simulink model "ACC_CarSim"  (Simulink 8.1)
settings: Solver=FixedStepDiscrete  StartTime=0.0  StopTime=100  FixedStep=0.001  MaxStep=0.001  RelTol=1e-3
PreLoadFcn:
  | Ts = 0.01;
undefined symbols (not defined in the file): DiscIntNeverNeededParam, sigbuilder_block
libraries: simulink x4, Solver_SF x1
settings Model: Creator=IVDL_Mola  LastModifiedBy=IVDL
settings DataIOCC: SignalLoggingSaveFormat=Dataset
settings OptimizationCC: ExpressionDepthLimit=128
settings DebuggingCC: FcnCallInpInsideContextMsg=EnableAllAsError  StateNameClashWarn=none
settings GRTTargetCC: CodeReplacementLibrary=None  CombineOutputUpdateFcns=on  CPPClassGenCompliant=on  GRTInterface=off

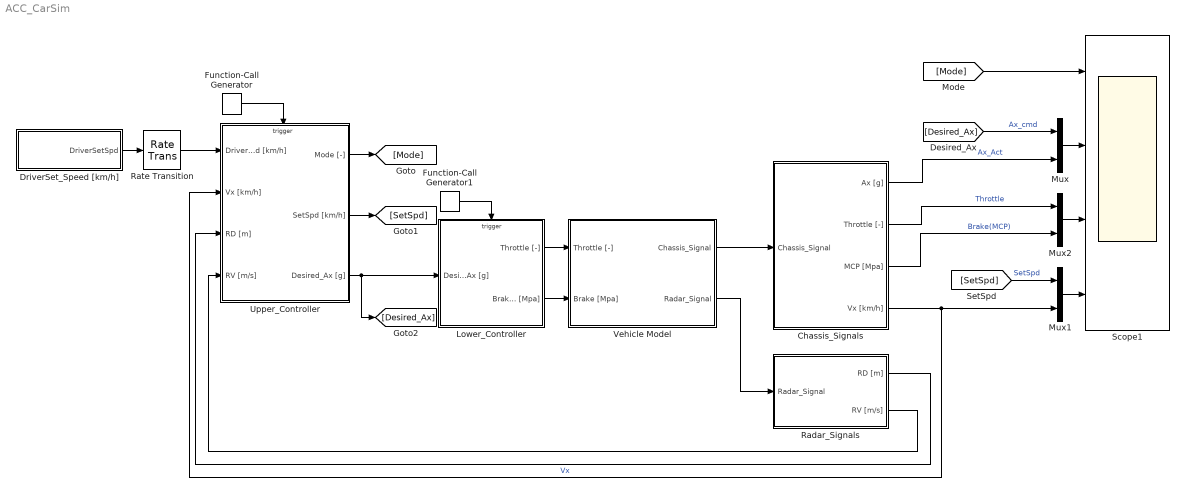
== system ACC_CarSim ==
  Chassis_Signals : Subsystem  SystemSampleTime=Ts
      settings: MinAlgLoopOccurrences=on
  DriverSet_Speed [km/h] : Subsystem  Tag=STV Subsys  LoadFcn=sigbuilder_block('load');  StartFcn=sigbuilder_block('start');  StopFcn=sigbuilder_block('stop');  ClipboardFcn=sigbuilder_block('clipboard');  mask(Sigbuilder block){}
      mask help: Simulink:masks:SigbuilderBlock_MD
      mask init:
      | if ~strcmp(get_param(bdroot(gcbh),'SimulationStatus'),'stopped') tuvar = sigbuilder_block('maskInit'); end
      settings: CopyFcn=sigbuilder_block('copy');  DeleteFcn=sigbuilder_block('delete');  ModelCloseFcn=sigbuilder_block('modelClose');  PreSaveFcn=sigbuilder_block('preSave');  PauseFcn=sigbuilder_block('pause');  ContinueFcn=sigbuilder_block('continue');  NameChangeFcn=sigbuilder_block('namechange');  OpenFcn=sigbuilder_block('open',[361.5 171.75 518.25 401.25 ]);  CloseFcn=sigbuilder_block('close');
      mask Display: plot(0, 0, 100, 100,[2, 2, 32, 32, 2], [68, 8, 8, 68, 68],[32, 2], [38, 38], [32, 19, 2],[53, 60, 44], [32, 17, 17, 2],[16, 16, 31, 31]);txt = getActiveGroup(gcbh);text(2, 100, txt,'verticalAlignment', 'top');
  Function-Call Generator : simulink/Ports & Subsystems/Function-Call Generator  sample_time=Ts  numberOfIterations=1
  Function-Call Generator1 : simulink/Ports & Subsystems/Function-Call Generator  sample_time=Ts  numberOfIterations=1
  Lower_Controller : Subsystem
  Mux : Mux  Inputs=2
  Mux1 : Mux  Inputs=2
  Mux2 : Mux  Inputs=2
  Radar_Signals : Subsystem  SystemSampleTime=Ts
  Rate Transition : RateTransition
  Scope1 : Scope  NumInputPorts=4
      settings: ShowLegends=on  TimeRange=100  YMin=0~-0.4~0~55  YMax=1~0.3~1.3~115
  Upper_Controller : Subsystem
  Vehicle Model : Subsystem
  wires:
  Upper_Controller/3(Desired_Ax [g]) -> [Desired_Ax], Lower_Controller/1(Desired_Ax [g])
  Lower_Controller/2(Brake [Mpa]) -> Vehicle Model/2(Brake [Mpa])
  Function-Call Generator/1 -> Upper_Controller/Trigger
  Function-Call Generator1/1 -> Lower_Controller/Trigger
  Vehicle Model/1(Chassis_Signal) -> Chassis_Signals/1(Chassis_Signal)
  Vehicle Model/2(Radar_Signal) -> Radar_Signals/1(Radar_Signal)
  Radar_Signals/2(RV [m/s]) -> Upper_Controller/4(RV [m/s])
  Radar_Signals/1(RD [m]) -> Upper_Controller/3(RD [m])
  DriverSet_Speed [km/h]/1(DriverSetSpd) -> Rate Transition/1
  Upper_Controller/1(Mode [-]) -> [Mode]
  Upper_Controller/2(SetSpd [km/h]) -> [SetSpd]
  Mux/1 -> Scope1/2
  Chassis_Signals/4(Vx [km/h]) -> Mux1/2, Upper_Controller/2(Vx [km/h])  "Vx"
  [Mode] -> Scope1/1
  [SetSpd] -> Mux1/1  "SetSpd"
  [Desired_Ax] -> Mux/1  "Ax_cmd"
  Mux2/1 -> Scope1/3
  Mux1/1 -> Scope1/4
  Chassis_Signals/1(Ax [g]) -> Mux/2  "Ax_Act"
  Chassis_Signals/2(Throttle [-]) -> Mux2/1  "Throttle"
  Chassis_Signals/3(MCP [Mpa]) -> Mux2/2  "Brake(MCP)"
  Rate Transition/1 -> Upper_Controller/1(Driver_SetSpd [km/h])
  Lower_Controller/1(Throttle [-]) -> Vehicle Model/1(Throttle [-])

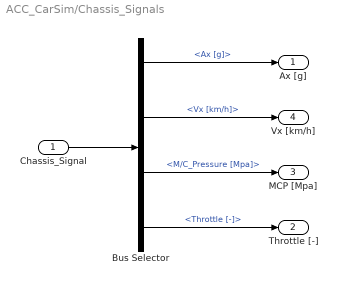
== system ACC_CarSim/Chassis_Signals ==
  Chassis_Signal : Inport
  Bus Selector : BusSelector  OutputSignals=Ax [g],Vx [km/h],M/C_Pressure [Mpa],Throttle [-]
  Ax [g] : Outport
  Throttle [-] : Outport  Port=2
  MCP [Mpa] : Outport  Port=3
  Vx [km/h] : Outport  Port=4
  wires:
  Bus Selector/2 -> Vx [km/h]/1  "<Vx [km/h]>"
  Bus Selector/1 -> Ax [g]/1  "<Ax [g]>"
  Chassis_Signal/1 -> Bus Selector/1
  Bus Selector/3 -> MCP [Mpa]/1  "<M/C_Pressure [Mpa]>"
  Bus Selector/4 -> Throttle [-]/1  "<Throttle [-]>"

== system ACC_CarSim/DriverSet_Speed [km/h] ==
  Demux : Demux  Tag=STV Demux  Outputs=1
  FromWs : FromWorkspace  Tag=STV FromWs  VariableName=tuvar  SampleTime=0  SigBuilderData=DataTag0  VnvData=DataTag1
      SigBuilderData=|
      | common.afterFinalStr = 'Extrapolate'
      | common.sampleTime = 0
      | dataSet.timeRange = [0 100]
      | dataSet.name = 'Group 1'
      | sbobj.Groups.Name = 'Group 1'
      | sbobj.Groups.Signals.Name = 'DriverSetSpd'
      | sbobj.Groups.Signals.XData = [0 25 25 80 80 100]
      | sbobj.Groups.Signals.YData = [70 70 110 110 60 60]
      | sbobj.Groups.TimeRange = [0 100]
  DriverSetSpd : Outport  Tag=STV Outport
  wires:
  Demux/1 -> DriverSetSpd/1
  FromWs/1 -> Demux/1

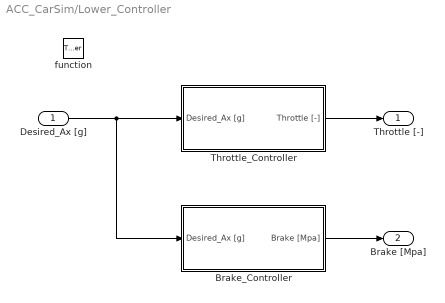
== system ACC_CarSim/Lower_Controller ==
  Desired_Ax [g] : Inport
  function : TriggerPort  TriggerType=function-call
  Brake_Controller : Subsystem
  Throttle_Controller : Subsystem
  Throttle [-] : Outport
  Brake [Mpa] : Outport  Port=2
  wires:
  Desired_Ax [g]/1 -> Brake_Controller/1(Desired_Ax [g]), Throttle_Controller/1(Desired_Ax [g])
  Throttle_Controller/1(Throttle [-]) -> Throttle [-]/1
  Brake_Controller/1(Brake [Mpa]) -> Brake [Mpa]/1

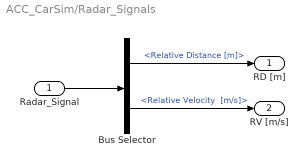
== system ACC_CarSim/Radar_Signals ==
  Radar_Signal : Inport
  Bus Selector : BusSelector  OutputSignals="Relative Distance [m],Relative Velocity  [m/s]"
  RD [m] : Outport
  RV [m/s] : Outport  Port=2
  wires:
  Radar_Signal/1 -> Bus Selector/1
  Bus Selector/1 -> RD [m]/1  "<Relative Distance [m]>"
  Bus Selector/2 -> RV [m/s]/1  "<Relative Velocity  [m/s]>"

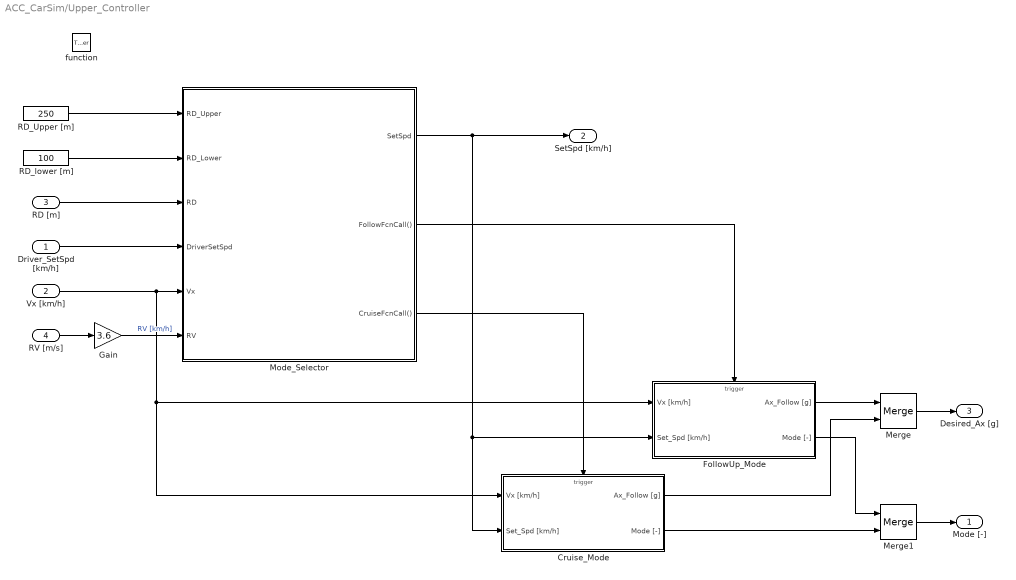
== system ACC_CarSim/Upper_Controller ==
  Driver_SetSpd [km/h] : Inport
  Vx [km/h] : Inport  Port=2
  RD [m] : Inport  Port=3
  RV [m/s] : Inport  Port=4
  function : TriggerPort  TriggerType=function-call
  Cruise_Mode : Subsystem  TreatAsAtomicUnit=on
  FollowUp_Mode : Subsystem  TreatAsAtomicUnit=on
  Gain : Gain  Gain=3.6
  Merge : Merge
  Merge1 : Merge
  Mode_Selector : Stateflow chart  TreatAsAtomicUnit=on
  RD_Upper [m] : Constant  Value=250
  RD_lower [m] : Constant  Value=100
  Mode [-] : Outport
  SetSpd [km/h] : Outport  Port=2
  Desired_Ax [g] : Outport  Port=3
  wires:
  RD_lower [m]/1 -> Mode_Selector/2(RD_Lower)
  RD_Upper [m]/1 -> Mode_Selector/1(RD_Upper)
  Driver_SetSpd [km/h]/1 -> Mode_Selector/4(DriverSetSpd)
  RD [m]/1 -> Mode_Selector/3(RD)
  Vx [km/h]/1 -> FollowUp_Mode/1(Vx [km/h]), Cruise_Mode/1(Vx [km/h]), Mode_Selector/5(Vx)
  RV [m/s]/1 -> Gain/1
  Gain/1 -> Mode_Selector/6(RV)  "RV [km/h]"
  Cruise_Mode/1(Ax_Follow [g]) -> Merge/2
  FollowUp_Mode/2(Mode [-]) -> Merge1/1
  Cruise_Mode/2(Mode [-]) -> Merge1/2
  Merge/1 -> Desired_Ax [g]/1
  Merge1/1 -> Mode [-]/1
  Mode_Selector/1(SetSpd) -> Cruise_Mode/2(Set_Spd [km/h]), FollowUp_Mode/2(Set_Spd [km/h]), SetSpd [km/h]/1
  Mode_Selector/2(FollowFcnCall()) -> FollowUp_Mode/Trigger
  Mode_Selector/3(CruiseFcnCall()) -> Cruise_Mode/Trigger
  FollowUp_Mode/1(Ax_Follow [g]) -> Merge/1

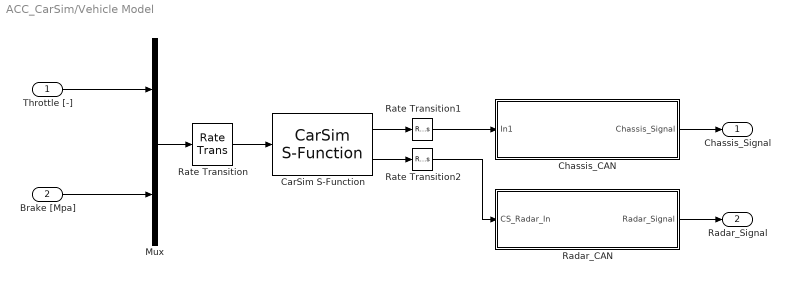
== system ACC_CarSim/Vehicle Model ==
  Throttle [-] : Inport
  Brake [Mpa] : Inport  Port=2
  CarSim S-Function : Solver_SF/CarSim S-Function  Priority=1  VehicleCode=i_i  SIMFILE=simfile
  Chassis_CAN : Subsystem
  Mux : Mux  Inputs=2
  Radar_CAN : Subsystem
  Rate Transition : RateTransition
  Rate Transition1 : RateTransition
  Rate Transition2 : RateTransition
  Chassis_Signal : Outport
  Radar_Signal : Outport  Port=2
  wires:
  Throttle [-]/1 -> Mux/1
  Radar_CAN/1(Radar_Signal) -> Radar_Signal/1
  Brake [Mpa]/1 -> Mux/2
  Mux/1 -> Rate Transition/1
  Chassis_CAN/1(Chassis_Signal) -> Chassis_Signal/1
  CarSim S-Function/1 -> Rate Transition1/1
  CarSim S-Function/2 -> Rate Transition2/1
  Rate Transition/1 -> CarSim S-Function/1
  Rate Transition1/1 -> Chassis_CAN/1(In1)
  Rate Transition2/1 -> Radar_CAN/1(CS_Radar_In)

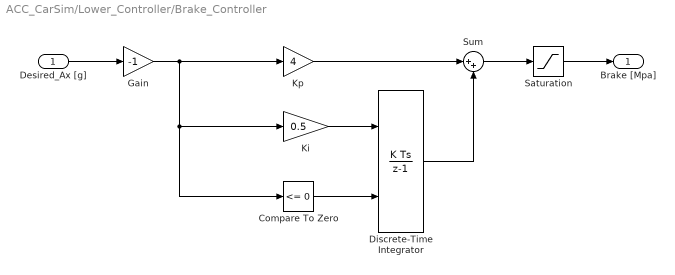
== system ACC_CarSim/Lower_Controller/Brake_Controller ==
  Desired_Ax [g] : Inport
  Compare To Zero : simulink/Logic and Bit Operations/Compare To Zero  relop=<=  OutDataTypeStr=boolean
  Discrete-Time Integrator : DiscreteIntegrator  ExternalReset=rising  SampleTime=-1  ICPrevOutput=DiscIntNeverNeededParam  ICPrevScaledInput=DiscIntNeverNeededParam
  Gain : Gain  Gain=-1
  Ki : Gain  Gain=0.5
  Kp : Gain  Gain=4
  Saturation : Saturate  UpperLimit=6  LowerLimit=0
  Sum : Sum  Inputs=|++
  Brake [Mpa] : Outport
  wires:
  Sum/1 -> Saturation/1
  Saturation/1 -> Brake [Mpa]/1
  Desired_Ax [g]/1 -> Gain/1
  Kp/1 -> Sum/1
  Ki/1 -> Discrete-Time Integrator/1
  Discrete-Time Integrator/1 -> Sum/2
  Gain/1 -> Compare To Zero/1, Ki/1, Kp/1
  Compare To Zero/1 -> Discrete-Time Integrator/2

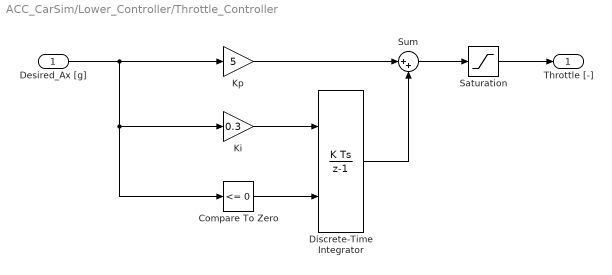
== system ACC_CarSim/Lower_Controller/Throttle_Controller ==
  Desired_Ax [g] : Inport
  Compare To Zero : simulink/Logic and Bit Operations/Compare To Zero  relop=<=  OutDataTypeStr=boolean
  Discrete-Time Integrator : DiscreteIntegrator  ExternalReset=rising  SampleTime=-1  ICPrevOutput=DiscIntNeverNeededParam  ICPrevScaledInput=DiscIntNeverNeededParam
  Ki : Gain  Gain=0.3
  Kp : Gain  Gain=5
  Saturation : Saturate  UpperLimit=0.7  LowerLimit=0
  Sum : Sum  Inputs=|++
  Throttle [-] : Outport
  wires:
  Sum/1 -> Saturation/1
  Saturation/1 -> Throttle [-]/1
  Desired_Ax [g]/1 -> Compare To Zero/1, Ki/1, Kp/1
  Kp/1 -> Sum/1
  Ki/1 -> Discrete-Time Integrator/1
  Compare To Zero/1 -> Discrete-Time Integrator/2
  Discrete-Time Integrator/1 -> Sum/2

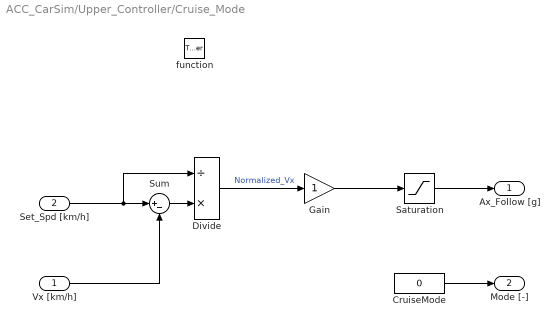
== system ACC_CarSim/Upper_Controller/Cruise_Mode ==
  Vx [km/h] : Inport
  Set_Spd [km/h] : Inport  Port=2
  function : TriggerPort  TriggerType=function-call
  CruiseMode : Constant  Value=0
  Divide : Product  Inputs=/*
  Gain : Gain
  Saturation : Saturate  UpperLimit=0.3  LowerLimit=-0.3
  Sum : Sum  Inputs=|+-
  Ax_Follow [g] : Outport
  Mode [-] : Outport  Port=2
  wires:
  Set_Spd [km/h]/1 -> Divide/1, Sum/1
  Vx [km/h]/1 -> Sum/2
  Sum/1 -> Divide/2
  Divide/1 -> Gain/1  "Normalized_Vx"
  Gain/1 -> Saturation/1
  Saturation/1 -> Ax_Follow [g]/1
  CruiseMode/1 -> Mode [-]/1

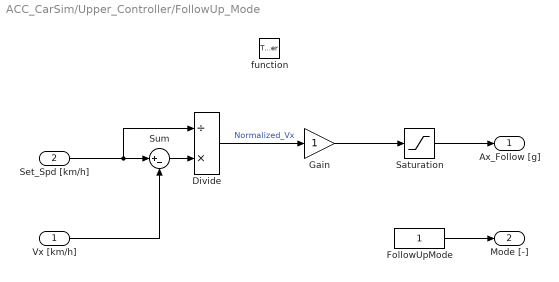
== system ACC_CarSim/Upper_Controller/FollowUp_Mode ==
  Vx [km/h] : Inport
  Set_Spd [km/h] : Inport  Port=2
  function : TriggerPort  TriggerType=function-call
  Divide : Product  Inputs=/*
  FollowUpMode : Constant
  Gain : Gain
  Saturation : Saturate  UpperLimit=0.4  LowerLimit=-0.4
  Sum : Sum  Inputs=|+-
  Ax_Follow [g] : Outport
  Mode [-] : Outport  Port=2
  wires:
  Set_Spd [km/h]/1 -> Divide/1, Sum/1
  Vx [km/h]/1 -> Sum/2
  Sum/1 -> Divide/2
  Divide/1 -> Gain/1  "Normalized_Vx"
  Gain/1 -> Saturation/1
  Saturation/1 -> Ax_Follow [g]/1
  FollowUpMode/1 -> Mode [-]/1

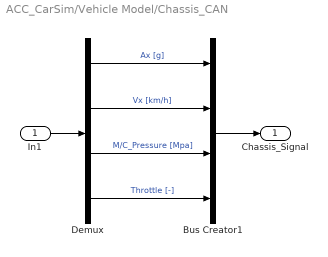
== system ACC_CarSim/Vehicle Model/Chassis_CAN ==
  In1 : Inport
  Bus Creator1 : BusCreator
  Demux : Demux
  Chassis_Signal : Outport
  wires:
  Demux/4 -> Bus Creator1/4  "Throttle [-]"
  Demux/3 -> Bus Creator1/3  "M/C_Pressure [Mpa]"
  Demux/2 -> Bus Creator1/2  "Vx [km/h]"
  Demux/1 -> Bus Creator1/1  "Ax [g]"
  In1/1 -> Demux/1
  Bus Creator1/1 -> Chassis_Signal/1

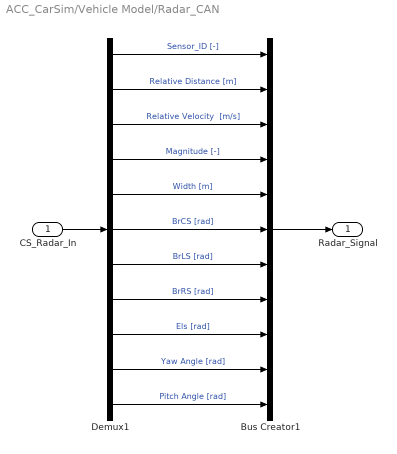
== system ACC_CarSim/Vehicle Model/Radar_CAN ==
  CS_Radar_In : Inport
  Bus Creator1 : BusCreator  Inputs=11
  Demux1 : Demux  Outputs=11
  Radar_Signal : Outport
  wires:
  Demux1/3 -> Bus Creator1/3  "Relative Velocity  [m/s]"
  Demux1/2 -> Bus Creator1/2  "Relative Distance [m]"
  Demux1/1 -> Bus Creator1/1  "Sensor_ID [-]"
  Demux1/8 -> Bus Creator1/8  "BrRS [rad]"
  Demux1/4 -> Bus Creator1/4  "Magnitude [-]"
  Demux1/7 -> Bus Creator1/7  "BrLS [rad]"
  Demux1/6 -> Bus Creator1/6  "BrCS [rad]"
  Demux1/10 -> Bus Creator1/10  "Yaw Angle [rad]"
  Demux1/11 -> Bus Creator1/11  "Pitch Angle [rad]"
  Demux1/5 -> Bus Creator1/5  "Width [m]"
  Demux1/9 -> Bus Creator1/9  "Els [rad]"
  CS_Radar_In/1 -> Demux1/1
  Bus Creator1/1 -> Radar_Signal/1

== stateflow chart Upper_Controller/Mode_Selector ==
  state Cruise_Mode
    du, en : TVSpd = RV+Vx;
    du : send(CruiseFcnCall)
    du : SetSpd = DriverSetSpd;
  state FollowUp_Mode
    du, en : TVSpd = RV+Vx;
    du : send(FollowFcnCall)
    du : SetSpd = TVSpd;
  (default) -> Cruise_Mode
  Cruise_Mode -> FollowUp_Mode : [(RD<=RD_Lower) & (DriverSetSpd >= TVSpd)]
  FollowUp_Mode -> Cruise_Mode : [(RD>RD_Upper) | (DriverSetSpd < TVSpd)]
  data: RD_Upper input double; RD_Lower input double; RD input double; DriverSetSpd input double; SetSpd output double; Vx input double; RV input double; TVSpd local double
  events: FollowFcnCall output FUNCTION_CALL_EVENT; CruiseFcnCall output FUNCTION_CALL_EVENT
